simulink model "Meta_atom_two_sphere_Newtons_cradle_simulation"  (R2024a)
settings: Solver=VariableStepAuto  StartTime=0.0  StopTime=5*0.3172  RelTol=1e-5
values from neighbouring files (symbols this model uses):
  c = 0    [Model_v3.m]
  cr = 0    [Code_to_set_initial_conditions_for_the_time_series_simulation.m]
  k = E*Rh^2/(2*R)    (= 9650000)    [Model_v3.m]
  kg = m*g/L    (= 0.874171340815)    [Model_v3.m]
  kr = mr*wr^2    [Code_to_generate_data_for_surface_plots.m]    (also in Code_to_set_initial_conditions_for_the_time_series_simulation.m = Omega*mr*(2*k/m))
  m = rho*(4/3)*pi*R^3-rho*(4/3)*pi*(R-Rh)^3    (= 0.00891102284215)    [Model_v3.m]
  mr = m    (= 0.00891102284215)    [Model_v3.m]
  R = 0.01    [Model_v3.m]
libraries: simulink x1
settings Model: Creator=Simon  LastModifiedBy=Simon Pope
settings SolverCC: AlgebraicLoopSolver=TrustRegion
settings DataIOCC: ReturnWorkspaceOutputsName=Sim_out
settings DebuggingCC: UnconnectedInputMsg=warning  UnconnectedOutputMsg=warning  UnconnectedLineMsg=warning
settings ModelReferenceCC: EnableRefExpFcnMdlSchedulingChecks=on
settings RTWCC: GPUComputeCapability=3.5  DLArmComputeVersion=19.05

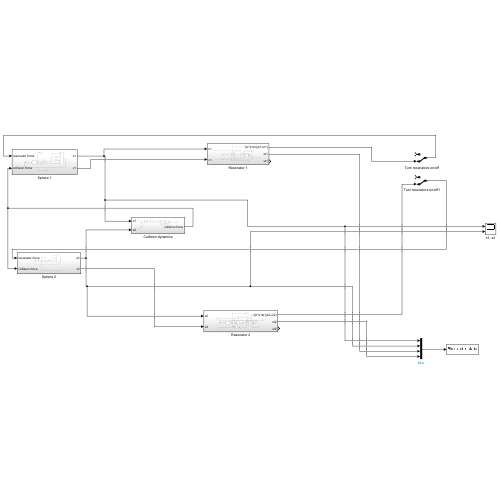
[thumbnail: Simulink's stored preview of the top-level diagram]
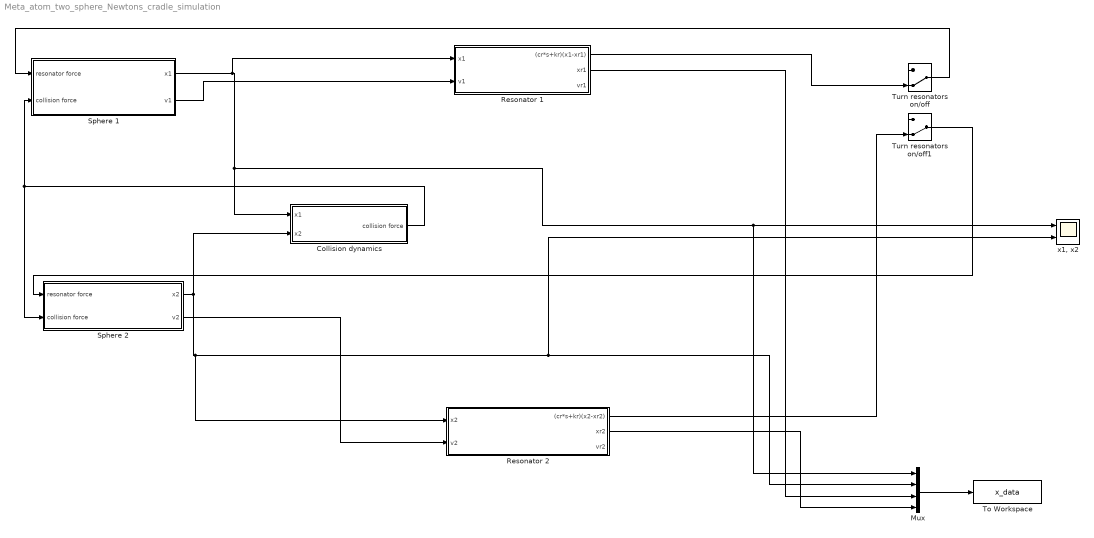
== system Meta_atom_two_sphere_Newtons_cradle_simulation ==
  Collision dynamics : Subsystem
  Mux : Mux
  Resonator 1 : Subsystem
  Resonator 2 : Subsystem
  Sphere 1 : Subsystem
  Sphere 2 : Subsystem
  To Workspace : ToWorkspace  VariableName=x_data  SaveFormat=Structure With Time  SampleTime=-1
  Turn resonators on/off : ManualSwitch  CurrentSetting=0
  Turn resonators on/off1 : ManualSwitch  CurrentSetting=0
  "x1, x2" : Scope  NumInputPorts=2
  wires:
  Resonator 1/2(xr1) -> Mux/3
  Resonator 1/1((cr*s+kr)(x1-xr1)) -> Turn resonators on/off/2
  Resonator 2/2(xr2) -> Mux/4
  Resonator 2/1((cr*s+kr)(x2-xr2)) -> Turn resonators on/off1/2
  Mux/1 -> To Workspace/1
  Sphere 1/1(x1) -> Resonator 1/1(x1), Collision dynamics/1(x1), Mux/1, "x1, x2"/1
  Turn resonators on/off/1 -> Sphere 1/1(resonator force)
  Sphere 1/2(v1) -> Resonator 1/2(v1)
  Sphere 2/1(x2) -> Collision dynamics/2(x2), Resonator 2/1(x2), Mux/2, "x1, x2"/2
  Turn resonators on/off1/1 -> Sphere 2/1(resonator force)
  Sphere 2/2(v2) -> Resonator 2/2(v2)
  Collision dynamics/1(collision force) -> Sphere 2/2(collision force), Sphere 1/2(collision force)

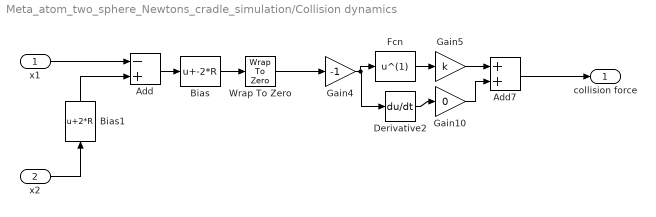
== system Meta_atom_two_sphere_Newtons_cradle_simulation/Collision dynamics ==
  x1 : Inport
  x2 : Inport  Port=2
  Add : Sum  Inputs=-+
  Add7 : Sum
  Bias : Bias  Bias=-2*R  SaturateOnIntegerOverflow=off
  Bias1 : Bias  Bias=2*R  SaturateOnIntegerOverflow=off
  Derivative2 : Derivative
  Fcn : Fcn  Expr=u^(1)
  Gain10 : Gain  Gain=0
  Gain4 : Gain  Gain=-1
  Gain5 : Gain  Gain=k
  Wrap To Zero : simulink/Discontinuities/Wrap To Zero  Threshold=0
  collision force : Outport
  wires:
  Wrap To Zero/1 -> Gain4/1
  Gain10/1 -> Add7/2
  Gain5/1 -> Add7/1
  Add/1 -> Bias/1
  Fcn/1 -> Gain5/1
  Bias1/1 -> Add/2
  Gain4/1 -> Derivative2/1, Fcn/1
  Derivative2/1 -> Gain10/1
  Bias/1 -> Wrap To Zero/1
  x1/1 -> Add/1
  Add7/1 -> collision force/1
  x2/1 -> Bias1/1

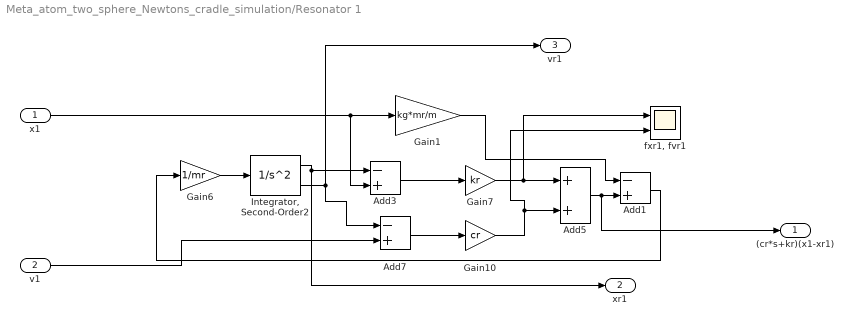
== system Meta_atom_two_sphere_Newtons_cradle_simulation/Resonator 1 ==
  x1 : Inport
  v1 : Inport  Port=2
  Add1 : Sum  Inputs=-+
  Add3 : Sum  Inputs=-+
  Add5 : Sum
  Add7 : Sum  Inputs=-+
  Gain1 : Gain  Gain=kg*mr/m
  Gain10 : Gain  Gain=cr
  Gain6 : Gain  Gain=1/mr
  Gain7 : Gain  Gain=kr
  "Integrator, Second-Order2" : SecondOrderIntegrator  ICX=x1r_initial  ICDXDT=dx1r_initial
  "fxr1, fvr1" : Scope  NumInputPorts=2
  (cr*s+kr)(x1-xr1) : Outport
  xr1 : Outport  Port=2
  vr1 : Outport  Port=3
  wires:
  "Integrator, Second-Order2"/2 -> Add7/1, vr1/1
  Gain7/1 -> Add5/1, "fxr1, fvr1"/1
  Add3/1 -> Gain7/1
  Gain6/1 -> "Integrator, Second-Order2"/1
  "Integrator, Second-Order2"/1 -> xr1/1, Add3/1
  x1/1 -> Add3/2, Gain1/1
  Add7/1 -> Gain10/1
  v1/1 -> Add7/2
  Gain10/1 -> "fxr1, fvr1"/2, Add5/2
  Add5/1 -> Add1/2, (cr*s+kr)(x1-xr1)/1
  Gain1/1 -> Add1/1
  Add1/1 -> Gain6/1

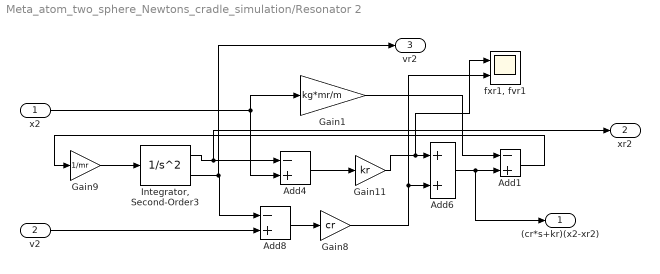
== system Meta_atom_two_sphere_Newtons_cradle_simulation/Resonator 2 ==
  x2 : Inport
  v2 : Inport  Port=2
  Add1 : Sum  Inputs=-+
  Add4 : Sum  Inputs=-+
  Add6 : Sum
  Add8 : Sum  Inputs=-+
  Gain1 : Gain  Gain=kg*mr/m
  Gain11 : Gain  Gain=kr
  Gain8 : Gain  Gain=cr
  Gain9 : Gain  Gain=1/mr
  "Integrator, Second-Order3" : SecondOrderIntegrator  ICX=0
  "fxr1, fvr1" : Scope  NumInputPorts=2
  (cr*s+kr)(x2-xr2) : Outport
  xr2 : Outport  Port=2
  vr2 : Outport  Port=3
  wires:
  Gain11/1 -> "fxr1, fvr1"/1, Add6/1
  Add4/1 -> Gain11/1
  Gain9/1 -> "Integrator, Second-Order3"/1
  "Integrator, Second-Order3"/2 -> vr2/1, Add8/1
  Add8/1 -> Gain8/1
  Gain8/1 -> Add6/2, "fxr1, fvr1"/2
  "Integrator, Second-Order3"/1 -> xr2/1, Add4/1
  x2/1 -> Gain1/1, Add4/2
  v2/1 -> Add8/2
  Add6/1 -> Add1/2, (cr*s+kr)(x2-xr2)/1
  Gain1/1 -> Add1/1
  Add1/1 -> Gain9/1

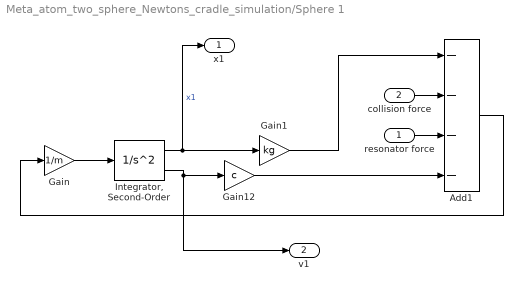
== system Meta_atom_two_sphere_Newtons_cradle_simulation/Sphere 1 ==
  resonator force : Inport
  collision force : Inport  Port=2
  Add1 : Sum  Inputs=----
  Gain : Gain  Gain=1/m
  Gain1 : Gain  Gain=kg
  Gain12 : Gain  Gain=c
  "Integrator, Second-Order" : SecondOrderIntegrator  ICX=x1_initial  ICDXDT=dx1_initial
  x1 : Outport
  v1 : Outport  Port=2
  wires:
  Add1/1 -> Gain/1
  "Integrator, Second-Order"/2 -> v1/1, Gain12/1
  resonator force/1 -> Add1/3
  Gain/1 -> "Integrator, Second-Order"/1
  Gain12/1 -> Add1/4
  Gain1/1 -> Add1/1
  "Integrator, Second-Order"/1 -> x1/1, Gain1/1  "x1"
  collision force/1 -> Add1/2

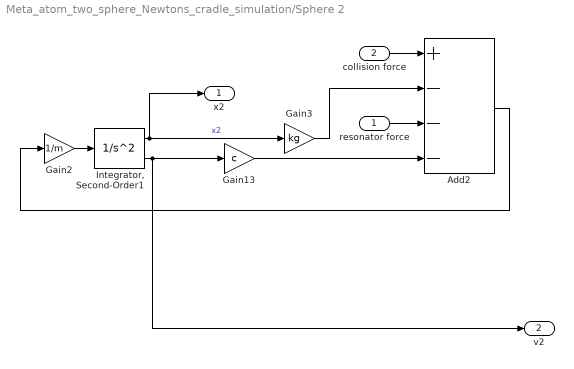
== system Meta_atom_two_sphere_Newtons_cradle_simulation/Sphere 2 ==
  resonator force : Inport
  collision force : Inport  Port=2
  Add2 : Sum  Inputs=+---
  Gain13 : Gain  Gain=c
  Gain2 : Gain  Gain=1/m
  Gain3 : Gain  Gain=kg
  "Integrator, Second-Order1" : SecondOrderIntegrator  ICX=0
  x2 : Outport
  v2 : Outport  Port=2
  wires:
  Gain2/1 -> "Integrator, Second-Order1"/1
  collision force/1 -> Add2/1
  Gain13/1 -> Add2/4
  Add2/1 -> Gain2/1
  "Integrator, Second-Order1"/2 -> v2/1, Gain13/1
  Gain3/1 -> Add2/2
  "Integrator, Second-Order1"/1 -> x2/1, Gain3/1  "x2"
  resonator force/1 -> Add2/3
